simulink model "signal_bourre"  (R2020a)
settings: Solver=VariableStepAuto  StartTime=0.0  StopTime=Tsim  RelTol=1e-3
values from neighbouring files (symbols this model uses):
  Te = 1/Fe    (= 3.125e-06)    [projet.m]
settings Model: Creator=imbergam  LastModifiedBy=imbergam

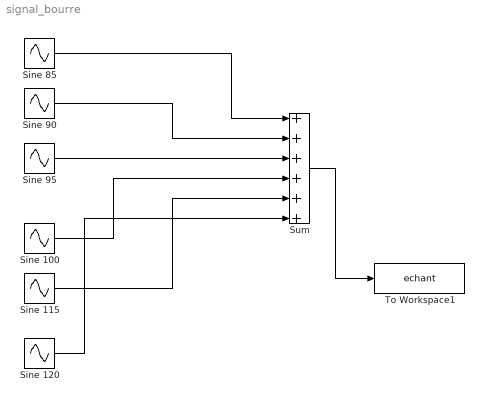
== system signal_bourre ==
  Sine 100 : Sin  Frequency=2*pi*100e3  SampleTime=0
  Sine 115 : Sin  Frequency=2*pi*115015.9  SampleTime=0
  Sine 120 : Sin  Frequency=2*pi*120e3  SampleTime=0
  Sine 85 : Sin  Frequency=2*pi*85005.9  SampleTime=0
  Sine 90 : Sin  Frequency=2*pi*90e3  SampleTime=0
  Sine 95 : Sin  Frequency=2*pi*94986.8  SampleTime=0
  Sum : Sum  Inputs=++++++
  To Workspace1 : ToWorkspace  VariableName=echant  SaveFormat=Timeseries  SampleTime=Te
  wires:
  Sine 85/1 -> Sum/1
  Sine 95/1 -> Sum/3
  Sine 115/1 -> Sum/5
  Sum/1 -> To Workspace1/1
  Sine 90/1 -> Sum/2
  Sine 100/1 -> Sum/4
  Sine 120/1 -> Sum/6
